simulink model "output_mux_core"  (R2013a)
settings: Solver=ode45  StartTime=0.0  StopTime=10.0  RelTol=1e-3
libraries: xbsIndex_r4 x496, casper_library_misc x1
(part 1 of 2)
settings Model: Creator=jack  LastModifiedBy=jack
settings OptimizationCC: ExpressionDepthLimit=2147483647

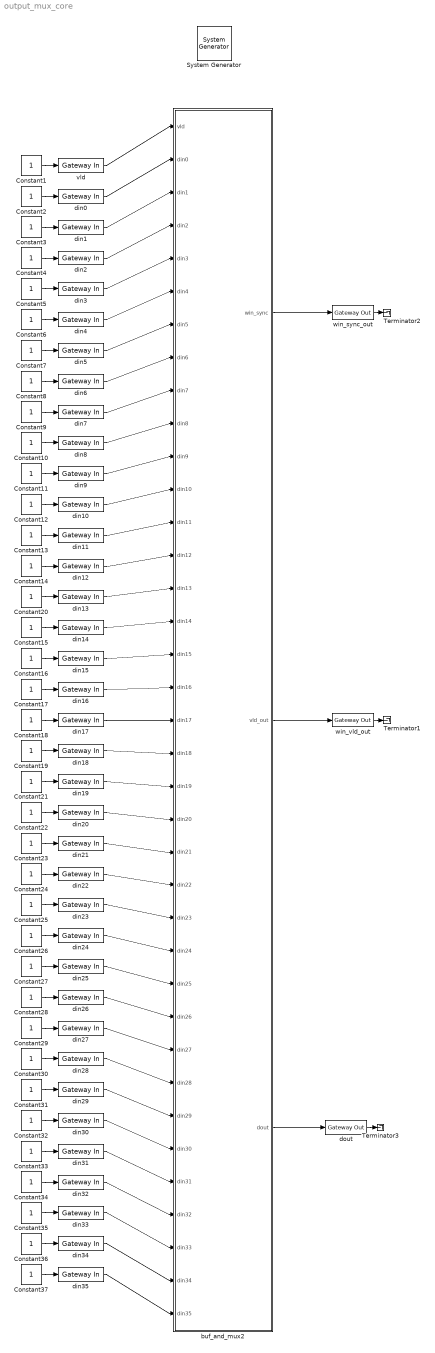
== system output_mux_core ==
  " System Generator" : xbsIndex_r4/ System Generator  Tag=genX  xilinxfamily=virtex6  part=xc6vsx475t  speed=-1  package=ff1759  synthesis_tool=XST  clock_wrapper=Clock Enables  directory=./output_mux_core  proj_type=Project Navigator  Synth_file=XST Defaults  Impl_file=ISE Defaults  testbench=off  simulink_period=1  sysclk_period=3.2  dcm_input_clock_period=10  incr_netlist=off  trim_vbits=Everywhere in SubSystem  dbl_ovrd=According to Block Masks  core_generation=According to Block Masks  run_coregen=off  deprecated_control=off  eval_field=0  block_type=sysgen
  Constant{1..37} (37 alike) : Constant
  Terminator1 : Terminator
  Terminator2 : Terminator
  Terminator3 : Terminator
  buf_and_mux2 : Subsystem  mask{bram_depth=10}
      mask prompts: bram_depth "bram depth (2^?)"
  din{0..35} (36 alike) : xbsIndex_r4/Gateway In  gui_display_data_type=Fixed-point  arith_type=Unsigned  n_bits=64  bin_pt=0  preci_type=Single  exp_width=8  frac_width=24  quantization="Round  (unbiased: +/- Inf)"  overflow=Saturate  period=1  dbl_ovrd=off  timing_constraint=None  locs_specified=off  LOCs={}  UseAsADC=off  ADCChannel='1'  inherit_from_input=off  hdl_port=on  block_type=gatewayin
  dout : xbsIndex_r4/Gateway Out  inherit_from_input=off  hdl_port=on  timing_constraint=None  locs_specified=off  LOCs={}  UseAsDAC=off  DACChannel='1'  block_type=gatewayout
  vld : xbsIndex_r4/Gateway In  gui_display_data_type=Boolean  arith_type=Boolean  n_bits=16  bin_pt=14  preci_type=Single  exp_width=8  frac_width=24  quantization="Round  (unbiased: +/- Inf)"  overflow=Saturate  period=1  dbl_ovrd=off  timing_constraint=None  locs_specified=off  LOCs={}  UseAsADC=off  ADCChannel='1'  inherit_from_input=off  hdl_port=on  block_type=gatewayin
  win_sync_out : xbsIndex_r4/Gateway Out  inherit_from_input=off  hdl_port=on  timing_constraint=None  locs_specified=off  LOCs={}  UseAsDAC=off  DACChannel='1'  block_type=gatewayout
  win_vld_out : xbsIndex_r4/Gateway Out  inherit_from_input=off  hdl_port=on  timing_constraint=None  locs_specified=off  LOCs={}  UseAsDAC=off  DACChannel='1'  block_type=gatewayout
  wires:
  Constant1/1 -> vld/1
  Constant2/1 -> din0/1
  win_sync_out/1 -> Terminator2/1
  vld/1 -> buf_and_mux2/1(vld)
  din0/1 -> buf_and_mux2/2(din0)
  dout/1 -> Terminator3/1
  Constant3/1 -> din1/1
  Constant4/1 -> din2/1
  Constant5/1 -> din3/1
  Constant6/1 -> din4/1
  Constant7/1 -> din5/1
  Constant8/1 -> din6/1
  Constant9/1 -> din7/1
  Constant10/1 -> din8/1
  Constant11/1 -> din9/1
  Constant12/1 -> din10/1
  Constant13/1 -> din11/1
  Constant14/1 -> din12/1
  Constant20/1 -> din13/1
  din5/1 -> buf_and_mux2/7(din5)
  din13/1 -> buf_and_mux2/15(din13)
  din7/1 -> buf_and_mux2/9(din7)
  din3/1 -> buf_and_mux2/5(din3)
  din12/1 -> buf_and_mux2/14(din12)
  din11/1 -> buf_and_mux2/13(din11)
  din4/1 -> buf_and_mux2/6(din4)
  din1/1 -> buf_and_mux2/3(din1)
  din8/1 -> buf_and_mux2/10(din8)
  din10/1 -> buf_and_mux2/12(din10)
  din9/1 -> buf_and_mux2/11(din9)
  din2/1 -> buf_and_mux2/4(din2)
  din6/1 -> buf_and_mux2/8(din6)
  Constant15/1 -> din14/1
  Constant16/1 -> din15/1
  Constant17/1 -> din16/1
  Constant18/1 -> din17/1
  Constant19/1 -> din18/1
  Constant21/1 -> din19/1
  Constant22/1 -> din20/1
  Constant23/1 -> din21/1
  Constant24/1 -> din22/1
  Constant25/1 -> din23/1
  Constant26/1 -> din24/1
  Constant27/1 -> din25/1
  Constant28/1 -> din26/1
  Constant29/1 -> din27/1
  Constant30/1 -> din28/1
  Constant31/1 -> din29/1
  Constant32/1 -> din30/1
  Constant33/1 -> din31/1
  Constant34/1 -> din32/1
  Constant35/1 -> din33/1
  Constant36/1 -> din34/1
  Constant37/1 -> din35/1
  din21/1 -> buf_and_mux2/23(din21)
  din27/1 -> buf_and_mux2/29(din27)
  din31/1 -> buf_and_mux2/33(din31)
  din33/1 -> buf_and_mux2/35(din33)
  din25/1 -> buf_and_mux2/27(din25)
  din34/1 -> buf_and_mux2/36(din34)
  din20/1 -> buf_and_mux2/22(din20)
  din35/1 -> buf_and_mux2/37(din35)
  din24/1 -> buf_and_mux2/26(din24)
  din16/1 -> buf_and_mux2/18(din16)
  din18/1 -> buf_and_mux2/20(din18)
  din23/1 -> buf_and_mux2/25(din23)
  din29/1 -> buf_and_mux2/31(din29)
  din30/1 -> buf_and_mux2/32(din30)
  din19/1 -> buf_and_mux2/21(din19)
  din14/1 -> buf_and_mux2/16(din14)
  din28/1 -> buf_and_mux2/30(din28)
  din17/1 -> buf_and_mux2/19(din17)
  din22/1 -> buf_and_mux2/24(din22)
  din26/1 -> buf_and_mux2/28(din26)
  din15/1 -> buf_and_mux2/17(din15)
  din32/1 -> buf_and_mux2/34(din32)
  buf_and_mux2/1(win_sync) -> win_sync_out/1
  buf_and_mux2/3(dout) -> dout/1
  win_vld_out/1 -> Terminator1/1
  buf_and_mux2/2(vld_out) -> win_vld_out/1

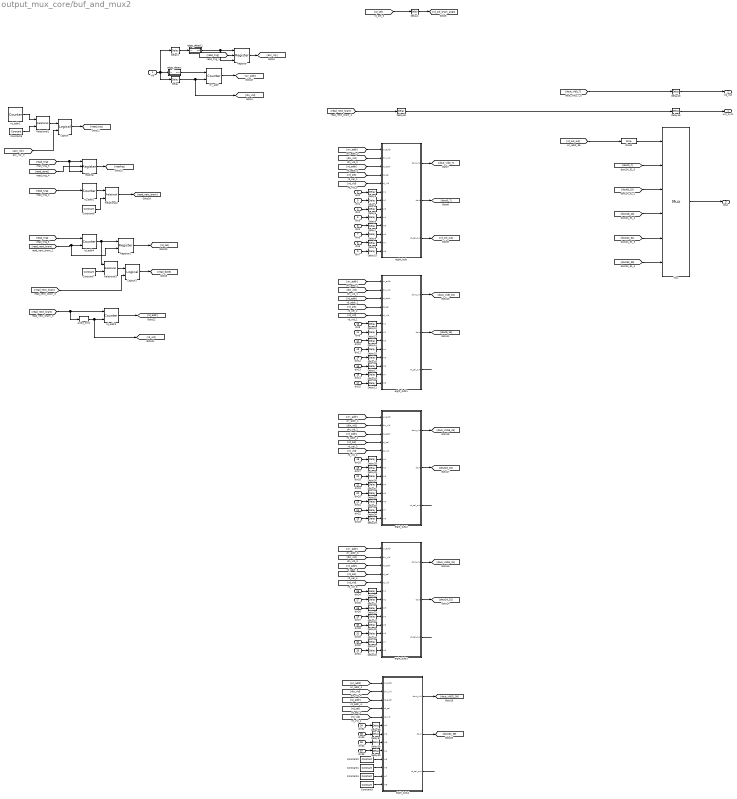
== system output_mux_core/buf_and_mux2 ==
  vld : Inport
  din0 : Inport  Port=2
  din1 : Inport  Port=3
  din2 : Inport  Port=4
  din3 : Inport  Port=5
  din4 : Inport  Port=6
  din5 : Inport  Port=7
  din6 : Inport  Port=8
  din7 : Inport  Port=9
  din8 : Inport  Port=10
  din9 : Inport  Port=11
  din10 : Inport  Port=12
  din11 : Inport  Port=13
  din12 : Inport  Port=14
  din13 : Inport  Port=15
  din14 : Inport  Port=16
  din15 : Inport  Port=17
  din16 : Inport  Port=18
  din17 : Inport  Port=19
  din18 : Inport  Port=20
  din19 : Inport  Port=21
  din20 : Inport  Port=22
  din21 : Inport  Port=23
  din22 : Inport  Port=24
  din23 : Inport  Port=25
  din24 : Inport  Port=26
  din25 : Inport  Port=27
  din26 : Inport  Port=28
  din27 : Inport  Port=29
  din28 : Inport  Port=30
  din29 : Inport  Port=31
  din30 : Inport  Port=32
  din31 : Inport  Port=33
  din32 : Inport  Port=34
  din33 : Inport  Port=35
  din34 : Inport  Port=36
  din35 : Inport  Port=37
  Constant{1..4} (4 alike) : xbsIndex_r4/Constant  const=0  gui_display_data_type=Fixed-point  arith_type=Unsigned  n_bits=64  bin_pt=0  preci_type=Single  exp_width=8  frac_width=24  explicit_period=on  period=1  equ=P=C  opselect=C  inp2=PCIN>>17  opr=+  inp1=P  carry=CIN  dbl_ovrd=off  block_type=constant
  Constant5 : xbsIndex_r4/Constant  const=0  gui_display_data_type=Fixed-point  arith_type=Unsigned  n_bits=bram_depth + 6 + 2  bin_pt=0  preci_type=Single  exp_width=8  frac_width=24  explicit_period=on  period=1  equ=P=C  opselect=C  inp2=PCIN>>17  opr=+  inp1=P  carry=CIN  dbl_ovrd=off  block_type=constant
  Constant6 : xbsIndex_r4/Constant  const=0  gui_display_data_type=Fixed-point  arith_type=Unsigned  n_bits=bram_depth +1  bin_pt=0  preci_type=Single  exp_width=8  frac_width=24  explicit_period=on  period=1  equ=P=C  opselect=C  inp2=PCIN>>17  opr=+  inp1=P  carry=CIN  dbl_ovrd=off  block_type=constant
  Constant7 : xbsIndex_r4/Constant  const=35  gui_display_data_type=Fixed-point  arith_type=Unsigned  n_bits=6  bin_pt=0  preci_type=Single  exp_width=8  frac_width=24  explicit_period=on  period=1  equ=P=C  opselect=C  inp2=PCIN>>17  opr=+  inp1=P  carry=CIN  dbl_ovrd=off  block_type=constant
  Delay{,1,3..34,36..39} (38 alike) : xbsIndex_r4/Delay  rst=off  infoeditControl=Selection of Reset will increase slice count due to use of real FFs and instead of SRLs  en=off  latency=1  dbl_ovrd=off  reg_retiming=off  block_type=delay
  Delay2 : xbsIndex_r4/Delay  rst=off  infoeditControl=Selection of Reset will increase slice count due to use of real FFs and instead of SRLs  en=off  latency=3  dbl_ovrd=off  reg_retiming=off  block_type=delay
  Delay43 : xbsIndex_r4/Delay  rst=off  infoeditControl=Selection of Reset will increase slice count due to use of real FFs and instead of SRLs  en=off  latency=2  dbl_ovrd=off  reg_retiming=off  block_type=delay
  Delay45 : xbsIndex_r4/Delay  rst=off  infoeditControl=Selection of Reset will increase slice count due to use of real FFs and instead of SRLs  en=off  latency=7  dbl_ovrd=off  reg_retiming=on  block_type=delay
  Delay46 : xbsIndex_r4/Delay  rst=off  infoeditControl=Selection of Reset will increase slice count due to use of real FFs and instead of SRLs  en=off  latency=2  dbl_ovrd=off  reg_retiming=off  block_type=delay
  Logical : xbsIndex_r4/Logical  logical_function=AND  inputs=2  en=off  latency=0  precision=Full  arith_type=Unsigned  n_bits=16  bin_pt=0  align_bp=on  dbl_ovrd=off  block_type=logical
  Logical1 : xbsIndex_r4/Logical  logical_function=AND  inputs=2  en=off  latency=0  precision=Full  arith_type=Unsigned  n_bits=16  bin_pt=0  align_bp=on  dbl_ovrd=off  block_type=logical
  Mux : xbsIndex_r4/Mux  inputs=5  en=off  latency=2  precision=Full  arith_type=Unsigned  n_bits=16  bin_pt=14  quantization=Truncate  overflow=Wrap  dbl_ovrd=off  block_type=mux
  Register : xbsIndex_r4/Register  init=0  rst=on  en=on  dbl_ovrd=off  block_type=register
  Register1 : xbsIndex_r4/Register  init=0  rst=off  en=on  dbl_ovrd=off  block_type=register
  Relational1 : xbsIndex_r4/Relational  mode=a=b  en=off  latency=1  dbl_ovrd=off  block_type=relational
  Relational2 : xbsIndex_r4/Relational  mode=a=b  en=off  latency=0  dbl_ovrd=off  block_type=relational
  Relational3 : xbsIndex_r4/Relational  mode=a=b  en=off  latency=0  dbl_ovrd=off  block_type=relational
  Slice2 : xbsIndex_r4/Slice  nbits=3  boolean_output=off  mode=Lower Bit Location + Width  bit1=0  base1=MSB of Input  bit0=3  base0=LSB of Input  dbl_ovrd=off  block_type=slice
  edge_detect : Subsystem  AncestorBlock=casper_library_misc/edge_detect  mask(edge_detect){edge=Rising, polarity=Active High, x_in=[0 0.08 0.08 0.16 0.16 0.24 0.24 0.32 0.32 0.4], y_in=[-1 -1  1  1  1  1  1  1  1  1], x_out=[0.6 0.68 0.68 0.76 0.76 0.84 0.84 0.92 0.92 1], y_out=[-1 -1  1  1 -1 -1 -1 -1 -1 -1]}
      mask prompts: edge "Edge Type"; polarity "Output Polarity"; x_in "Input X Positions"; y_in "Input Y Positions"; x_out "Output X Positions"; y_out "Output Y Positions"
      mask help: Output is active for one-cycle after each edge of the specified type (i.e. rising, falling or both).
      mask init:
      | edge_detect_init(gcb,...
      |     'edge',edge,...
      |     'polarity',polarity,...
      |     'x_in',x_in,...
      |     'x_out',x_out,...
      |     'y_in',y_in,...
      |     'y_out',y_out);
      | 
      | x_in_num=str2num(getfield(getfield(get_param(gcb,'UserData'),'parameters'),'x_in'));
      | x_out_num=str2num(getfield(getfield(get_param(gcb,'UserData'),'parameters'),'x_out'));
      | y_in_num=str2num(getfield(getfield(get_param(gcb,'UserData'),'parameters'),'y_in'));
      | y_out_num=str2num(getfield(getfield(get_param(gcb,'UserData'),'parameters'),'y_out'));
      settings: AttributesFormatString=|
      | rising edges
      | active high
      mask Help: Output is active for one-cycle after each edge of the specified type (i.e. rising, falling, or both).  Latency is zero.
      mask TypeOptions edge: Rising | Falling | Both
      mask TypeOptions polarity: Active High | Active Low
      mask Display:
      | plot(x_in_num,0.5+y_in_num*0.2);
      | plot(x_out_num,0.5+y_out_num*0.2);
  edge_detect1 : Subsystem  AncestorBlock=casper_library_misc/edge_detect  mask(edge_detect){edge=Falling, polarity=Active High, x_in=[0 0.08 0.08 0.16 0.16 0.24 0.24 0.32 0.32 0.4], y_in=[-1 -1  1  1  1  1  1  1  1  1], x_out=[0.6 0.68 0.68 0.76 0.76 0.84 0.84 0.92 0.92 1], y_out=[-1 -1  1  1 -1 -1 -1 -1 -1 -1]}
      mask prompts: edge "Edge Type"; polarity "Output Polarity"; x_in "Input X Positions"; y_in "Input Y Positions"; x_out "Output X Positions"; y_out "Output Y Positions"
      mask help: Output is active for one-cycle after each edge of the specified type (i.e. rising, falling or both).
      mask init: same as output_mux_core/buf_and_mux2/edge_detect
      settings: AttributesFormatString=|
      | falling edges
      | active high
      mask Help: Output is active for one-cycle after each edge of the specified type (i.e. rising, falling, or both).  Latency is zero.
      mask TypeOptions edge: Rising | Falling | Both
      mask TypeOptions polarity: Active High | Active Low
      mask Display:
      | plot(x_in_num,0.5+y_in_num*0.2);
      | plot(x_out_num,0.5+y_out_num*0.2);
  eight_bufs : Subsystem
  eight_bufs1 : Subsystem
  eight_bufs2 : Subsystem
  eight_bufs3 : Subsystem
  eight_bufs4 : Subsystem
  pulse_ext1 : casper_library_misc/pulse_ext  pulse_len=2^bram_depth
  rd_addr1 : xbsIndex_r4/Counter  cnt_type=Free Running  cnt_to=Inf  operation=Up  start_count=0  cnt_by_val=1  arith_type=Unsigned  n_bits=bram_depth + 6 + 2  bin_pt=0  load_pin=off  rst=off  en=off  explicit_period=on  period=1  dbl_ovrd=off  use_behavioral_HDL=off  implementation=Fabric  block_type=counter
  rd_addr2 : xbsIndex_r4/Counter  cnt_type=Count Limited  cnt_to=2^bram_depth  operation=Up  start_count=0  cnt_by_val=1  arith_type=Unsigned  n_bits=bram_depth + 1  bin_pt=0  load_pin=off  rst=on  en=off  explicit_period=on  period=1  dbl_ovrd=off  use_behavioral_HDL=off  implementation=DSP48  block_type=counter
  rd_addr3 : xbsIndex_r4/Counter  cnt_type=Free Running  cnt_to=Inf  operation=Up  start_count=0  cnt_by_val=1  arith_type=Unsigned  n_bits=bram_depth  bin_pt=0  load_pin=off  rst=on  en=on  explicit_period=on  period=1  dbl_ovrd=off  use_behavioral_HDL=off  implementation=Fabric  block_type=counter
  rd_addr4 : xbsIndex_r4/Counter  cnt_type=Free Running  cnt_to=Inf  operation=Up  start_count=0  cnt_by_val=1  arith_type=Unsigned  n_bits=6  bin_pt=0  load_pin=off  rst=on  en=on  explicit_period=on  period=1  dbl_ovrd=off  use_behavioral_HDL=off  implementation=Fabric  block_type=counter
  reading : xbsIndex_r4/Register  init=0  rst=on  en=on  dbl_ovrd=off  block_type=register
  wr_addr : xbsIndex_r4/Counter  cnt_type=Free Running  cnt_to=Inf  operation=Up  start_count=0  cnt_by_val=1  arith_type=Unsigned  n_bits=bram_depth  bin_pt=0  load_pin=off  rst=on  en=on  explicit_period=on  period=1  dbl_ovrd=off  use_behavioral_HDL=off  implementation=DSP48  block_type=counter
  win_sync : Outport
  vld_out : Outport  Port=2
  dout : Outport  Port=3
  wires:
  Register1/1 -> [rd_sel]
  rd_addr4/1 -> Relational3/1, Register1/1
  [read_next_bram] -> rd_addr4/2, Register1/2
  [read_trig] -> rd_addr4/1
  rd_addr3/1 -> [rd_addr]
  pulse_ext1/1 -> rd_addr3/2, [rd_vld]
  [read_next_bram] -> rd_addr3/1, pulse_ext1/1
  [read_done] -> reading/2
  reading/1 -> [reading]
  [read_trig] -> reading/1, reading/3
  Relational2/1 -> [read_next_bram]
  Constant6/1 -> Relational2/2
  rd_addr2/1 -> Relational2/1
  [read_trig] -> rd_addr2/1
  Logical/1 -> [read_trig]
  [acc_rdy] -> Logical/2
  Relational1/1 -> Logical/1
  Constant5/1 -> Relational1/2
  rd_addr1/1 -> Relational1/1
  [read_trig] -> Register/2
  Register/1 -> [acc_rdy]
  Constant4/1 -> eight_bufs4/12(In7)
  Constant3/1 -> eight_bufs4/13(In8)
  Constant1/1 -> eight_bufs4/11(In6)
  Constant2/1 -> eight_bufs4/10(In5)
  Mux/1 -> dout/1
  Delay46/1 -> win_sync/1
  Delay45/1 -> Delay46/1
  [read_next_bram] -> Delay45/1
  Delay43/1 -> vld_out/1
  [dout_vld0_7] -> Delay43/1
  [dout32_39] -> Mux/6
  [dout24_31] -> Mux/5
  [dout8_15] -> Mux/3
  [dout16_23] -> Mux/4
  [dout0_7] -> Mux/2
  eight_bufs4/3(rd_sel_out) -> ?
  eight_bufs4/2(dout) -> [dout32_39]
  eight_bufs4/1(dout_vld) -> [dout_vld32_39]
  Delay39/1 -> eight_bufs4/9(In4)
  Delay38/1 -> eight_bufs4/8(In3)
  Delay37/1 -> eight_bufs4/7(In2)
  Delay36/1 -> eight_bufs4/6(In1)
  [wr_addr] -> eight_bufs4/1(wr_addr)
  [rd_vld] -> eight_bufs4/5(rd_vld)
  [rd_sel] -> eight_bufs4/4(rd_sel)
  [rd_addr] -> eight_bufs4/3(rd_addr)
  [din_vld] -> eight_bufs4/2(din_vld)
  din35/1 -> Delay39/1
  din34/1 -> Delay38/1
  din33/1 -> Delay37/1
  din32/1 -> Delay36/1
  eight_bufs3/3(rd_sel_out) -> ?
  eight_bufs3/2(dout) -> [dout24_31]
  eight_bufs3/1(dout_vld) -> [dout_vld24_31]
  Delay20/1 -> eight_bufs3/13(In8)
  Delay27/1 -> eight_bufs3/12(In7)
  Delay26/1 -> eight_bufs3/11(In6)
  Delay25/1 -> eight_bufs3/10(In5)
  Delay24/1 -> eight_bufs3/9(In4)
  Delay23/1 -> eight_bufs3/8(In3)
  Delay22/1 -> eight_bufs3/7(In2)
  Delay21/1 -> eight_bufs3/6(In1)
  [wr_addr] -> eight_bufs3/1(wr_addr)
  [rd_vld] -> eight_bufs3/5(rd_vld)
  [rd_sel] -> eight_bufs3/4(rd_sel)
  [rd_addr] -> eight_bufs3/3(rd_addr)
  [din_vld] -> eight_bufs3/2(din_vld)
  din31/1 -> Delay20/1
  din30/1 -> Delay27/1
  din29/1 -> Delay26/1
  din28/1 -> Delay25/1
  din27/1 -> Delay24/1
  din26/1 -> Delay23/1
  din25/1 -> Delay22/1
  din24/1 -> Delay21/1
  eight_bufs2/3(rd_sel_out) -> ?
  eight_bufs2/2(dout) -> [dout16_23]
  eight_bufs2/1(dout_vld) -> [dout_vld16_23]
  Delay19/1 -> eight_bufs2/13(In8)
  Delay34/1 -> eight_bufs2/12(In7)
  Delay33/1 -> eight_bufs2/11(In6)
  Delay32/1 -> eight_bufs2/10(In5)
  Delay31/1 -> eight_bufs2/9(In4)
  Delay30/1 -> eight_bufs2/8(In3)
  Delay29/1 -> eight_bufs2/7(In2)
  Delay28/1 -> eight_bufs2/6(In1)
  [wr_addr] -> eight_bufs2/1(wr_addr)
  [rd_vld] -> eight_bufs2/5(rd_vld)
  [rd_sel] -> eight_bufs2/4(rd_sel)
  [rd_addr] -> eight_bufs2/3(rd_addr)
  [din_vld] -> eight_bufs2/2(din_vld)
  din23/1 -> Delay19/1
  din22/1 -> Delay34/1
  din21/1 -> Delay33/1
  din20/1 -> Delay32/1
  din19/1 -> Delay31/1
  din18/1 -> Delay30/1
  din17/1 -> Delay29/1
  din16/1 -> Delay28/1
  eight_bufs1/3(rd_sel_out) -> ?
  eight_bufs1/2(dout) -> [dout8_15]
  eight_bufs1/1(dout_vld) -> [dout_vld8_15]
  Delay11/1 -> eight_bufs1/13(In8)
  Delay18/1 -> eight_bufs1/12(In7)
  Delay17/1 -> eight_bufs1/11(In6)
  Delay16/1 -> eight_bufs1/10(In5)
  Delay15/1 -> eight_bufs1/9(In4)
  Delay14/1 -> eight_bufs1/8(In3)
  Delay13/1 -> eight_bufs1/7(In2)
  Delay12/1 -> eight_bufs1/6(In1)
  [wr_addr] -> eight_bufs1/1(wr_addr)
  [rd_vld] -> eight_bufs1/5(rd_vld)
  [rd_sel] -> eight_bufs1/4(rd_sel)
  [rd_addr] -> eight_bufs1/3(rd_addr)
  [din_vld] -> eight_bufs1/2(din_vld)
  din15/1 -> Delay11/1
  din14/1 -> Delay18/1
  din13/1 -> Delay17/1
  din12/1 -> Delay16/1
  din11/1 -> Delay15/1
  din10/1 -> Delay14/1
  din9/1 -> Delay13/1
  din8/1 -> Delay12/1
  Slice2/1 -> Mux/1
  [rd_sel_out] -> Slice2/1
  eight_bufs/3(rd_sel_out) -> [rd_sel_out]
  eight_bufs/2(dout) -> [dout0_7]
  eight_bufs/1(dout_vld) -> [dout_vld0_7]
  Delay10/1 -> eight_bufs/13(In8)
  Delay9/1 -> eight_bufs/12(In7)
  Delay8/1 -> eight_bufs/11(In6)
  Delay7/1 -> eight_bufs/10(In5)
  Delay6/1 -> eight_bufs/9(In4)
  Delay5/1 -> eight_bufs/8(In3)
  Delay4/1 -> eight_bufs/7(In2)
  Delay3/1 -> eight_bufs/6(In1)
  [wr_addr] -> eight_bufs/1(wr_addr)
  [rd_vld] -> eight_bufs/5(rd_vld)
  [rd_sel] -> eight_bufs/4(rd_sel)
  [rd_addr] -> eight_bufs/3(rd_addr)
  [din_vld] -> eight_bufs/2(din_vld)
  din7/1 -> Delay10/1
  din6/1 -> Delay9/1
  din5/1 -> Delay8/1
  din4/1 -> Delay7/1
  din3/1 -> Delay6/1
  din2/1 -> Delay5/1
  din1/1 -> Delay4/1
  din0/1 -> Delay3/1
  Delay2/1 -> [rd_sel_bram_align]
  [rd_sel] -> Delay2/1
  Delay1/1 -> edge_detect1/1(in)
  edge_detect1/1(out) -> Register/1, Register/3
  wr_addr/1 -> [wr_addr]
  Delay/1 -> wr_addr/2, [din_vld]
  edge_detect/1(out) -> wr_addr/1
  vld/1 -> edge_detect/1(in), Delay/1, Delay1/1
  Constant7/1 -> Relational3/2
  Relational3/1 -> Logical1/1
  [read_next_bram] -> Logical1/2
  Logical1/1 -> [read_done]

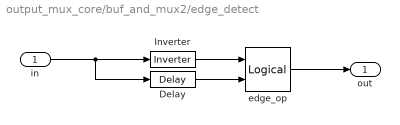
== system output_mux_core/buf_and_mux2/edge_detect ==
  in : Inport
  Delay : xbsIndex_r4/Delay  rst=off  infoeditControl=Selection of Reset will increase slice count due to use of real FFs and instead of SRLs  en=off  latency=1  dbl_ovrd=off  reg_retiming=off  block_type=delay
      settings: xl_area=[0, 0, 0, 0, 0, 0, 0]
  Inverter : xbsIndex_r4/Inverter  en=off  latency=0  dbl_ovrd=off  block_type=inv
      settings: xl_area=[0, 0, 0, 0, 0, 0, 0]
  edge_op : xbsIndex_r4/Logical  logical_function=NOR  inputs=2  en=off  latency=0  precision=Full  arith_type=Unsigned  n_bits=8  bin_pt=2  align_bp=on  dbl_ovrd=off  block_type=logical
      settings: xl_area=[0, 0, 0, 0, 0, 0, 0]
  out : Outport
  wires:
  Delay/1 -> edge_op/2
  in/1 -> Delay/1, Inverter/1
  edge_op/1 -> out/1
  Inverter/1 -> edge_op/1

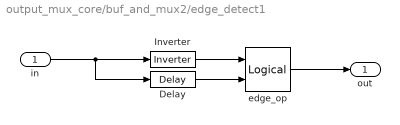
== system output_mux_core/buf_and_mux2/edge_detect1 ==
  in : Inport
  Delay : xbsIndex_r4/Delay  rst=off  infoeditControl=Selection of Reset will increase slice count due to use of real FFs and instead of SRLs  en=off  latency=1  dbl_ovrd=off  reg_retiming=off  block_type=delay
      settings: xl_area=[0, 0, 0, 0, 0, 0, 0]
  Inverter : xbsIndex_r4/Inverter  en=off  latency=0  dbl_ovrd=off  block_type=inv
      settings: xl_area=[0, 0, 0, 0, 0, 0, 0]
  edge_op : xbsIndex_r4/Logical  logical_function=AND  inputs=2  en=off  latency=0  precision=Full  arith_type=Unsigned  n_bits=8  bin_pt=2  align_bp=on  dbl_ovrd=off  block_type=logical
      settings: xl_area=[0, 0, 0, 0, 0, 0, 0]
  out : Outport
  wires:
  Inverter/1 -> edge_op/1
  edge_op/1 -> out/1
  in/1 -> Inverter/1, Delay/1
  Delay/1 -> edge_op/2

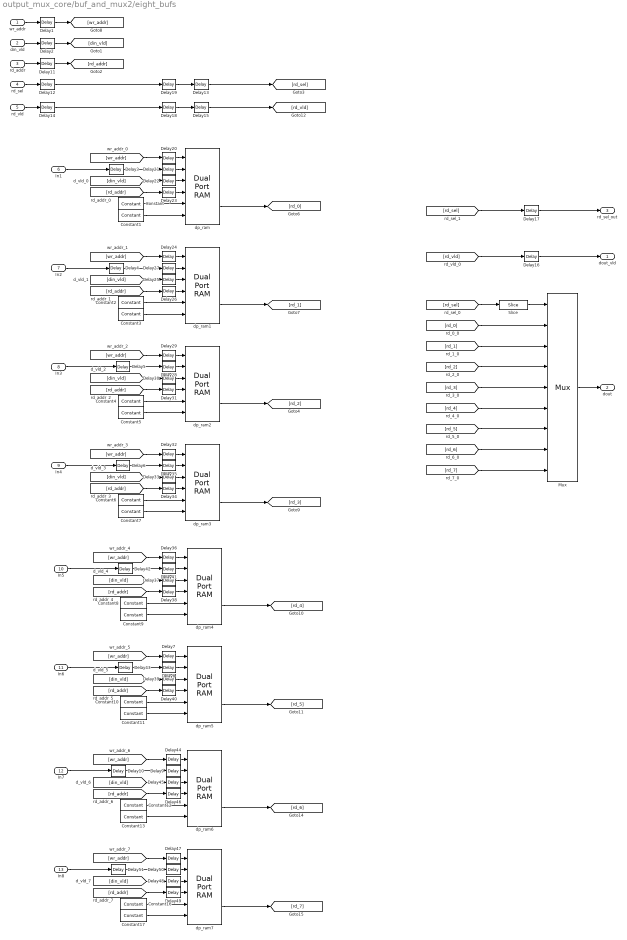
== system output_mux_core/buf_and_mux2/eight_bufs ==
  wr_addr : Inport
  din_vld : Inport  Port=2
  rd_addr : Inport  Port=3
  rd_sel : Inport  Port=4
  rd_vld : Inport  Port=5
  In1 : Inport  Port=6
  In2 : Inport  Port=7
  In3 : Inport  Port=8
  In4 : Inport  Port=9
  In5 : Inport  Port=10
  In6 : Inport  Port=11
  In7 : Inport  Port=12
  In8 : Inport  Port=13
  Constant{,2,4,6,8,10,12,16} (8 alike) : xbsIndex_r4/Constant  const=0  gui_display_data_type=Fixed-point  arith_type=Unsigned  n_bits=64  bin_pt=0  preci_type=Single  exp_width=8  frac_width=24  explicit_period=on  period=1  equ=P=C  opselect=C  inp2=PCIN>>17  opr=+  inp1=P  carry=CIN  dbl_ovrd=off  block_type=constant
  Constant{1,3,5,7,9,11,13,17} (8 alike) : xbsIndex_r4/Constant  const=0  gui_display_data_type=Boolean  arith_type=Boolean  n_bits=64  bin_pt=0  preci_type=Single  exp_width=8  frac_width=24  explicit_period=on  period=1  equ=P=C  opselect=C  inp2=PCIN>>17  opr=+  inp1=P  carry=CIN  dbl_ovrd=off  block_type=constant
  Delay{1..2,7,11..12,14,20,22..26,29..34,36..40,44..49} (29 alike) : xbsIndex_r4/Delay  rst=off  infoeditControl=Selection of Reset will increase slice count due to use of real FFs and instead of SRLs  en=off  latency=1  dbl_ovrd=off  reg_retiming=off  block_type=delay
  Delay{3..6,8..10,18..19,21,27..28,35,41..43,50..51} (18 alike) : xbsIndex_r4/Delay  rst=off  infoeditControl=Selection of Reset will increase slice count due to use of real FFs and instead of SRLs  en=off  latency=1  dbl_ovrd=off  reg_retiming=on  block_type=delay
  Delay13 : xbsIndex_r4/Delay  rst=off  infoeditControl=Selection of Reset will increase slice count due to use of real FFs and instead of SRLs  en=off  latency=3  dbl_ovrd=off  reg_retiming=on  block_type=delay
  Delay15 : xbsIndex_r4/Delay  rst=off  infoeditControl=Selection of Reset will increase slice count due to use of real FFs and instead of SRLs  en=off  latency=3  dbl_ovrd=off  reg_retiming=on  block_type=delay
  Delay16 : xbsIndex_r4/Delay  rst=off  infoeditControl=Selection of Reset will increase slice count due to use of real FFs and instead of SRLs  en=off  latency=2  dbl_ovrd=off  reg_retiming=off  block_type=delay
  Delay17 : xbsIndex_r4/Delay  rst=off  infoeditControl=Selection of Reset will increase slice count due to use of real FFs and instead of SRLs  en=off  latency=2  dbl_ovrd=off  reg_retiming=off  block_type=delay
  Mux : xbsIndex_r4/Mux  inputs=8  en=off  latency=2  precision=Full  arith_type=Unsigned  n_bits=16  bin_pt=14  quantization=Truncate  overflow=Wrap  dbl_ovrd=off  block_type=mux
  Slice : xbsIndex_r4/Slice  nbits=3  boolean_output=off  mode=Lower Bit Location + Width  bit1=0  base1=MSB of Input  bit0=0  base0=LSB of Input  dbl_ovrd=off  block_type=slice
  dp_ram{,1..7} (8 alike) : xbsIndex_r4/Dual Port RAM  depth=2^bram_depth  initVector=sin(pi*(0:15)/16)  distributed_mem=Block RAM  init_a=0  init_b=0  rst_a=off  rst_b=off  en_a=off  en_b=off  latency=3  write_mode_A=Read After Write  write_mode_B=Read After Write  dbl_ovrd=off  optimize=Speed  block_type=dpram
  dout_vld : Outport
  dout : Outport  Port=2
  rd_sel_out : Outport  Port=3
  wires:
  Slice/1 -> Mux/1
  Delay17/1 -> rd_sel_out/1
  [rd_sel] -> Delay17/1
  Delay16/1 -> dout_vld/1
  [rd_vld] -> Delay16/1
  Delay14/1 -> Delay18/1
  Delay15/1 -> [rd_vld]
  rd_vld/1 -> Delay14/1
  Mux/1 -> dout/1
  [rd_1] -> Mux/3
  [rd_2] -> Mux/4
  [rd_0] -> Mux/2
  [rd_5] -> Mux/7
  [rd_4] -> Mux/6
  [rd_sel] -> Slice/1
  [rd_7] -> Mux/9
  [rd_6] -> Mux/8
  [rd_3] -> Mux/5
  dp_ram7/2 -> [rd_7]
  dp_ram6/2 -> [rd_6]
  dp_ram5/2 -> [rd_5]
  dp_ram4/2 -> [rd_4]
  dp_ram3/2 -> [rd_3]
  dp_ram2/2 -> [rd_2]
  dp_ram1/2 -> [rd_1]
  dp_ram/2 -> [rd_0]
  Delay13/1 -> [rd_sel]
  Delay12/1 -> Delay19/1
  rd_sel/1 -> Delay12/1
  Delay11/1 -> [rd_addr]
  rd_addr/1 -> Delay11/1
  Delay2/1 -> [din_vld]
  din_vld/1 -> Delay2/1
  Delay1/1 -> [wr_addr]
  wr_addr/1 -> Delay1/1
  Constant1/1 -> dp_ram/6
  [wr_addr] -> Delay44/1
  Constant17/1 -> dp_ram7/6
  [wr_addr] -> Delay7/1
  [din_vld] -> Delay22/1
  [din_vld] -> Delay39/1
  Delay4/1 -> Delay27/1
  Delay51/1 -> Delay50/1
  [rd_addr] -> Delay46/1
  Constant7/1 -> dp_ram3/6
  In4/1 -> Delay6/1
  Constant11/1 -> dp_ram5/6
  Constant13/1 -> dp_ram6/6
  Delay42/1 -> Delay41/1
  [din_vld] -> Delay33/1
  Constant10/1 -> dp_ram5/5
  [rd_addr] -> Delay38/1
  Constant4/1 -> dp_ram2/5
  Constant12/1 -> dp_ram6/5
  Constant8/1 -> dp_ram4/5
  [din_vld] -> Delay30/1
  Delay43/1 -> Delay8/1
  [din_vld] -> Delay48/1
  [din_vld] -> Delay37/1
  [rd_addr] -> Delay40/1
  In1/1 -> Delay3/1
  [rd_addr] -> Delay34/1
  Delay10/1 -> Delay9/1
  [rd_addr] -> Delay31/1
  Delay5/1 -> Delay28/1
  [wr_addr] -> Delay47/1
  Constant16/1 -> dp_ram7/5
  In6/1 -> Delay43/1
  Constant6/1 -> dp_ram3/5
  Constant9/1 -> dp_ram4/6
  In3/1 -> Delay5/1
  In8/1 -> Delay51/1
  [wr_addr] -> Delay36/1
  [wr_addr] -> Delay29/1
  In7/1 -> Delay10/1
  Constant/1 -> dp_ram/5
  Constant5/1 -> dp_ram2/6
  [rd_addr] -> Delay49/1
  In5/1 -> Delay42/1
  [wr_addr] -> Delay32/1
  [wr_addr] -> Delay20/1
  [wr_addr] -> Delay24/1
  [rd_addr] -> Delay26/1
  In2/1 -> Delay4/1
  Constant2/1 -> dp_ram1/5
  Constant3/1 -> dp_ram1/6
  [din_vld] -> Delay25/1
  [din_vld] -> Delay45/1
  [rd_addr] -> Delay23/1
  Delay3/1 -> Delay21/1
  Delay18/1 -> Delay15/1
  Delay19/1 -> Delay13/1
  Delay20/1 -> dp_ram/1
  Delay21/1 -> dp_ram/2
  Delay22/1 -> dp_ram/3
  Delay23/1 -> dp_ram/4
  Delay24/1 -> dp_ram1/1
  Delay25/1 -> dp_ram1/3
  Delay26/1 -> dp_ram1/4
  Delay27/1 -> dp_ram1/2
  Delay28/1 -> dp_ram2/2
  Delay29/1 -> dp_ram2/1
  Delay30/1 -> dp_ram2/3
  Delay31/1 -> dp_ram2/4
  Delay32/1 -> dp_ram3/1
  Delay33/1 -> dp_ram3/3
  Delay34/1 -> dp_ram3/4
  Delay6/1 -> Delay35/1
  Delay35/1 -> dp_ram3/2
  Delay36/1 -> dp_ram4/1
  Delay37/1 -> dp_ram4/3
  Delay38/1 -> dp_ram4/4
  Delay7/1 -> dp_ram5/1
  Delay39/1 -> dp_ram5/3
  Delay40/1 -> dp_ram5/4
  Delay41/1 -> dp_ram4/2
  Delay8/1 -> dp_ram5/2
  Delay44/1 -> dp_ram6/1
  Delay45/1 -> dp_ram6/3
  Delay46/1 -> dp_ram6/4
  Delay47/1 -> dp_ram7/1
  Delay48/1 -> dp_ram7/3
  Delay49/1 -> dp_ram7/4
  Delay9/1 -> dp_ram6/2
  Delay50/1 -> dp_ram7/2

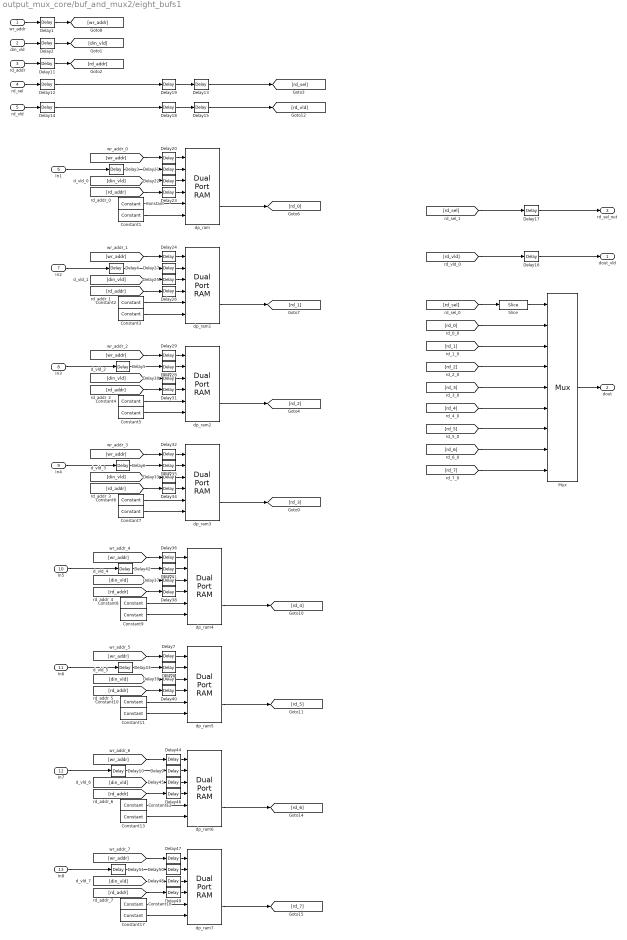
== system output_mux_core/buf_and_mux2/eight_bufs1 ==
  wr_addr : Inport
  din_vld : Inport  Port=2
  rd_addr : Inport  Port=3
  rd_sel : Inport  Port=4
  rd_vld : Inport  Port=5
  In1 : Inport  Port=6
  In2 : Inport  Port=7
  In3 : Inport  Port=8
  In4 : Inport  Port=9
  In5 : Inport  Port=10
  In6 : Inport  Port=11
  In7 : Inport  Port=12
  In8 : Inport  Port=13
  Constant{,2,4,6,8,10,12,16} (8 alike) : xbsIndex_r4/Constant  const=0  gui_display_data_type=Fixed-point  arith_type=Unsigned  n_bits=64  bin_pt=0  preci_type=Single  exp_width=8  frac_width=24  explicit_period=on  period=1  equ=P=C  opselect=C  inp2=PCIN>>17  opr=+  inp1=P  carry=CIN  dbl_ovrd=off  block_type=constant
  Constant{1,3,5,7,9,11,13,17} (8 alike) : xbsIndex_r4/Constant  const=0  gui_display_data_type=Boolean  arith_type=Boolean  n_bits=64  bin_pt=0  preci_type=Single  exp_width=8  frac_width=24  explicit_period=on  period=1  equ=P=C  opselect=C  inp2=PCIN>>17  opr=+  inp1=P  carry=CIN  dbl_ovrd=off  block_type=constant
  Delay{1..2,7,11..12,14,20,22..26,29..34,36..40,44..49} (29 alike) : xbsIndex_r4/Delay  rst=off  infoeditControl=Selection of Reset will increase slice count due to use of real FFs and instead of SRLs  en=off  latency=1  dbl_ovrd=off  reg_retiming=off  block_type=delay
  Delay{3..6,8..10,18..19,21,27..28,35,41..43,50..51} (18 alike) : xbsIndex_r4/Delay  rst=off  infoeditControl=Selection of Reset will increase slice count due to use of real FFs and instead of SRLs  en=off  latency=1  dbl_ovrd=off  reg_retiming=on  block_type=delay
  Delay13 : xbsIndex_r4/Delay  rst=off  infoeditControl=Selection of Reset will increase slice count due to use of real FFs and instead of SRLs  en=off  latency=3  dbl_ovrd=off  reg_retiming=on  block_type=delay
  Delay15 : xbsIndex_r4/Delay  rst=off  infoeditControl=Selection of Reset will increase slice count due to use of real FFs and instead of SRLs  en=off  latency=3  dbl_ovrd=off  reg_retiming=on  block_type=delay
  Delay16 : xbsIndex_r4/Delay  rst=off  infoeditControl=Selection of Reset will increase slice count due to use of real FFs and instead of SRLs  en=off  latency=2  dbl_ovrd=off  reg_retiming=off  block_type=delay
  Delay17 : xbsIndex_r4/Delay  rst=off  infoeditControl=Selection of Reset will increase slice count due to use of real FFs and instead of SRLs  en=off  latency=2  dbl_ovrd=off  reg_retiming=off  block_type=delay
  Mux : xbsIndex_r4/Mux  inputs=8  en=off  latency=2  precision=Full  arith_type=Unsigned  n_bits=16  bin_pt=14  quantization=Truncate  overflow=Wrap  dbl_ovrd=off  block_type=mux
  Slice : xbsIndex_r4/Slice  nbits=3  boolean_output=off  mode=Lower Bit Location + Width  bit1=0  base1=MSB of Input  bit0=0  base0=LSB of Input  dbl_ovrd=off  block_type=slice
  dp_ram{,1..7} (8 alike) : xbsIndex_r4/Dual Port RAM  depth=2^bram_depth  initVector=sin(pi*(0:15)/16)  distributed_mem=Block RAM  init_a=0  init_b=0  rst_a=off  rst_b=off  en_a=off  en_b=off  latency=3  write_mode_A=Read After Write  write_mode_B=Read After Write  dbl_ovrd=off  optimize=Speed  block_type=dpram
  dout_vld : Outport
  dout : Outport  Port=2
  rd_sel_out : Outport  Port=3
  wires:
  Delay50/1 -> dp_ram7/2
  Delay9/1 -> dp_ram6/2
  Delay49/1 -> dp_ram7/4
  Delay48/1 -> dp_ram7/3
  Delay47/1 -> dp_ram7/1
  Delay46/1 -> dp_ram6/4
  Delay45/1 -> dp_ram6/3
  Delay44/1 -> dp_ram6/1
  Delay8/1 -> dp_ram5/2
  Delay41/1 -> dp_ram4/2
  Delay40/1 -> dp_ram5/4
  Delay39/1 -> dp_ram5/3
  Delay7/1 -> dp_ram5/1
  Delay38/1 -> dp_ram4/4
  Delay37/1 -> dp_ram4/3
  Delay36/1 -> dp_ram4/1
  Delay35/1 -> dp_ram3/2
  Delay6/1 -> Delay35/1
  Delay34/1 -> dp_ram3/4
  Delay33/1 -> dp_ram3/3
  Delay32/1 -> dp_ram3/1
  Delay31/1 -> dp_ram2/4
  Delay30/1 -> dp_ram2/3
  Delay29/1 -> dp_ram2/1
  Delay28/1 -> dp_ram2/2
  Delay27/1 -> dp_ram1/2
  Delay26/1 -> dp_ram1/4
  Delay25/1 -> dp_ram1/3
  Delay24/1 -> dp_ram1/1
  Delay23/1 -> dp_ram/4
  Delay22/1 -> dp_ram/3
  Delay21/1 -> dp_ram/2
  Delay20/1 -> dp_ram/1
  Delay19/1 -> Delay13/1
  Delay18/1 -> Delay15/1
  Delay3/1 -> Delay21/1
  [rd_addr] -> Delay23/1
  [din_vld] -> Delay45/1
  [din_vld] -> Delay25/1
  Constant3/1 -> dp_ram1/6
  Constant2/1 -> dp_ram1/5
  In2/1 -> Delay4/1
  [rd_addr] -> Delay26/1
  [wr_addr] -> Delay24/1
  [wr_addr] -> Delay20/1
  [wr_addr] -> Delay32/1
  In5/1 -> Delay42/1
  [rd_addr] -> Delay49/1
  Constant5/1 -> dp_ram2/6
  Constant/1 -> dp_ram/5
  In7/1 -> Delay10/1
  [wr_addr] -> Delay29/1
  [wr_addr] -> Delay36/1
  In8/1 -> Delay51/1
  In3/1 -> Delay5/1
  Constant9/1 -> dp_ram4/6
  Constant6/1 -> dp_ram3/5
  In6/1 -> Delay43/1
  Constant16/1 -> dp_ram7/5
  [wr_addr] -> Delay47/1
  Delay5/1 -> Delay28/1
  [rd_addr] -> Delay31/1
  Delay10/1 -> Delay9/1
  [rd_addr] -> Delay34/1
  In1/1 -> Delay3/1
  [rd_addr] -> Delay40/1
  [din_vld] -> Delay37/1
  [din_vld] -> Delay48/1
  Delay43/1 -> Delay8/1
  [din_vld] -> Delay30/1
  Constant8/1 -> dp_ram4/5
  Constant12/1 -> dp_ram6/5
  Constant4/1 -> dp_ram2/5
  [rd_addr] -> Delay38/1
  Constant10/1 -> dp_ram5/5
  [din_vld] -> Delay33/1
  Delay42/1 -> Delay41/1
  Constant13/1 -> dp_ram6/6
  Constant11/1 -> dp_ram5/6
  In4/1 -> Delay6/1
  Constant7/1 -> dp_ram3/6
  [rd_addr] -> Delay46/1
  Delay51/1 -> Delay50/1
  Delay4/1 -> Delay27/1
  [din_vld] -> Delay39/1
  [din_vld] -> Delay22/1
  [wr_addr] -> Delay7/1
  Constant17/1 -> dp_ram7/6
  [wr_addr] -> Delay44/1
  Constant1/1 -> dp_ram/6
  wr_addr/1 -> Delay1/1
  Delay1/1 -> [wr_addr]
  din_vld/1 -> Delay2/1
  Delay2/1 -> [din_vld]
  rd_addr/1 -> Delay11/1
  Delay11/1 -> [rd_addr]
  rd_sel/1 -> Delay12/1
  Delay12/1 -> Delay19/1
  Delay13/1 -> [rd_sel]
  dp_ram/2 -> [rd_0]
  dp_ram1/2 -> [rd_1]
  dp_ram2/2 -> [rd_2]
  dp_ram3/2 -> [rd_3]
  dp_ram4/2 -> [rd_4]
  dp_ram5/2 -> [rd_5]
  dp_ram6/2 -> [rd_6]
  dp_ram7/2 -> [rd_7]
  [rd_3] -> Mux/5
  [rd_6] -> Mux/8
  [rd_7] -> Mux/9
  [rd_sel] -> Slice/1
  [rd_4] -> Mux/6
  [rd_5] -> Mux/7
  [rd_0] -> Mux/2
  [rd_2] -> Mux/4
  [rd_1] -> Mux/3
  Mux/1 -> dout/1
  rd_vld/1 -> Delay14/1
  Delay15/1 -> [rd_vld]
  Delay14/1 -> Delay18/1
  [rd_vld] -> Delay16/1
  Delay16/1 -> dout_vld/1
  [rd_sel] -> Delay17/1
  Delay17/1 -> rd_sel_out/1
  Slice/1 -> Mux/1

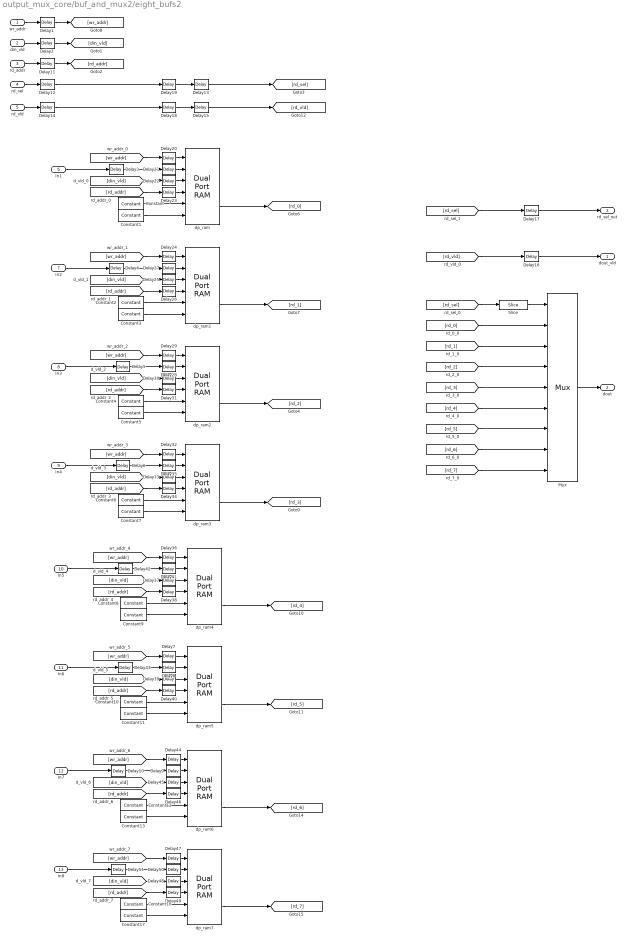
== system output_mux_core/buf_and_mux2/eight_bufs2 ==
  wr_addr : Inport
  din_vld : Inport  Port=2
  rd_addr : Inport  Port=3
  rd_sel : Inport  Port=4
  rd_vld : Inport  Port=5
  In1 : Inport  Port=6
  In2 : Inport  Port=7
  In3 : Inport  Port=8
  In4 : Inport  Port=9
  In5 : Inport  Port=10
  In6 : Inport  Port=11
  In7 : Inport  Port=12
  In8 : Inport  Port=13
  Constant{,2,4,6,8,10,12,16} (8 alike) : xbsIndex_r4/Constant  const=0  gui_display_data_type=Fixed-point  arith_type=Unsigned  n_bits=64  bin_pt=0  preci_type=Single  exp_width=8  frac_width=24  explicit_period=on  period=1  equ=P=C  opselect=C  inp2=PCIN>>17  opr=+  inp1=P  carry=CIN  dbl_ovrd=off  block_type=constant
  Constant{1,3,5,7,9,11,13,17} (8 alike) : xbsIndex_r4/Constant  const=0  gui_display_data_type=Boolean  arith_type=Boolean  n_bits=64  bin_pt=0  preci_type=Single  exp_width=8  frac_width=24  explicit_period=on  period=1  equ=P=C  opselect=C  inp2=PCIN>>17  opr=+  inp1=P  carry=CIN  dbl_ovrd=off  block_type=constant
  Delay{1..2,7,11..12,14,20,22..26,29..34,36..40,44..49} (29 alike) : xbsIndex_r4/Delay  rst=off  infoeditControl=Selection of Reset will increase slice count due to use of real FFs and instead of SRLs  en=off  latency=1  dbl_ovrd=off  reg_retiming=off  block_type=delay
  Delay{3..6,8..10,18..19,21,27..28,35,41..43,50..51} (18 alike) : xbsIndex_r4/Delay  rst=off  infoeditControl=Selection of Reset will increase slice count due to use of real FFs and instead of SRLs  en=off  latency=1  dbl_ovrd=off  reg_retiming=on  block_type=delay
  Delay13 : xbsIndex_r4/Delay  rst=off  infoeditControl=Selection of Reset will increase slice count due to use of real FFs and instead of SRLs  en=off  latency=3  dbl_ovrd=off  reg_retiming=on  block_type=delay
  Delay15 : xbsIndex_r4/Delay  rst=off  infoeditControl=Selection of Reset will increase slice count due to use of real FFs and instead of SRLs  en=off  latency=3  dbl_ovrd=off  reg_retiming=on  block_type=delay
  Delay16 : xbsIndex_r4/Delay  rst=off  infoeditControl=Selection of Reset will increase slice count due to use of real FFs and instead of SRLs  en=off  latency=2  dbl_ovrd=off  reg_retiming=off  block_type=delay
  Delay17 : xbsIndex_r4/Delay  rst=off  infoeditControl=Selection of Reset will increase slice count due to use of real FFs and instead of SRLs  en=off  latency=2  dbl_ovrd=off  reg_retiming=off  block_type=delay
  Mux : xbsIndex_r4/Mux  inputs=8  en=off  latency=2  precision=Full  arith_type=Unsigned  n_bits=16  bin_pt=14  quantization=Truncate  overflow=Wrap  dbl_ovrd=off  block_type=mux
  Slice : xbsIndex_r4/Slice  nbits=3  boolean_output=off  mode=Lower Bit Location + Width  bit1=0  base1=MSB of Input  bit0=0  base0=LSB of Input  dbl_ovrd=off  block_type=slice
  dp_ram{,1..7} (8 alike) : xbsIndex_r4/Dual Port RAM  depth=2^bram_depth  initVector=sin(pi*(0:15)/16)  distributed_mem=Block RAM  init_a=0  init_b=0  rst_a=off  rst_b=off  en_a=off  en_b=off  latency=3  write_mode_A=Read After Write  write_mode_B=Read After Write  dbl_ovrd=off  optimize=Speed  block_type=dpram
  dout_vld : Outport
  dout : Outport  Port=2
  rd_sel_out : Outport  Port=3
  wires:
  Slice/1 -> Mux/1
  Delay17/1 -> rd_sel_out/1
  [rd_sel] -> Delay17/1
  Delay16/1 -> dout_vld/1
  [rd_vld] -> Delay16/1
  Delay14/1 -> Delay18/1
  Delay15/1 -> [rd_vld]
  rd_vld/1 -> Delay14/1
  Mux/1 -> dout/1
  [rd_1] -> Mux/3
  [rd_2] -> Mux/4
  [rd_0] -> Mux/2
  [rd_5] -> Mux/7
  [rd_4] -> Mux/6
  [rd_sel] -> Slice/1
  [rd_7] -> Mux/9
  [rd_6] -> Mux/8
  [rd_3] -> Mux/5
  dp_ram7/2 -> [rd_7]
  dp_ram6/2 -> [rd_6]
  dp_ram5/2 -> [rd_5]
  dp_ram4/2 -> [rd_4]
  dp_ram3/2 -> [rd_3]
  dp_ram2/2 -> [rd_2]
  dp_ram1/2 -> [rd_1]
  dp_ram/2 -> [rd_0]
  Delay13/1 -> [rd_sel]
  Delay12/1 -> Delay19/1
  rd_sel/1 -> Delay12/1
  Delay11/1 -> [rd_addr]
  rd_addr/1 -> Delay11/1
  Delay2/1 -> [din_vld]
  din_vld/1 -> Delay2/1
  Delay1/1 -> [wr_addr]
  wr_addr/1 -> Delay1/1
  Constant1/1 -> dp_ram/6
  [wr_addr] -> Delay44/1
  Constant17/1 -> dp_ram7/6
  [wr_addr] -> Delay7/1
  [din_vld] -> Delay22/1
  [din_vld] -> Delay39/1
  Delay4/1 -> Delay27/1
  Delay51/1 -> Delay50/1
  [rd_addr] -> Delay46/1
  Constant7/1 -> dp_ram3/6
  In4/1 -> Delay6/1
  Constant11/1 -> dp_ram5/6
  Constant13/1 -> dp_ram6/6
  Delay42/1 -> Delay41/1
  [din_vld] -> Delay33/1
  Constant10/1 -> dp_ram5/5
  [rd_addr] -> Delay38/1
  Constant4/1 -> dp_ram2/5
  Constant12/1 -> dp_ram6/5
  Constant8/1 -> dp_ram4/5
  [din_vld] -> Delay30/1
  Delay43/1 -> Delay8/1
  [din_vld] -> Delay48/1
  [din_vld] -> Delay37/1
  [rd_addr] -> Delay40/1
  In1/1 -> Delay3/1
  [rd_addr] -> Delay34/1
  Delay10/1 -> Delay9/1
  [rd_addr] -> Delay31/1
  Delay5/1 -> Delay28/1
  [wr_addr] -> Delay47/1
  Constant16/1 -> dp_ram7/5
  In6/1 -> Delay43/1
  Constant6/1 -> dp_ram3/5
  Constant9/1 -> dp_ram4/6
  In3/1 -> Delay5/1
  In8/1 -> Delay51/1
  [wr_addr] -> Delay36/1
  [wr_addr] -> Delay29/1
  In7/1 -> Delay10/1
  Constant/1 -> dp_ram/5
  Constant5/1 -> dp_ram2/6
  [rd_addr] -> Delay49/1
  In5/1 -> Delay42/1
  [wr_addr] -> Delay32/1
  [wr_addr] -> Delay20/1
  [wr_addr] -> Delay24/1
  [rd_addr] -> Delay26/1
  In2/1 -> Delay4/1
  Constant2/1 -> dp_ram1/5
  Constant3/1 -> dp_ram1/6
  [din_vld] -> Delay25/1
  [din_vld] -> Delay45/1
  [rd_addr] -> Delay23/1
  Delay3/1 -> Delay21/1
  Delay18/1 -> Delay15/1
  Delay19/1 -> Delay13/1
  Delay20/1 -> dp_ram/1
  Delay21/1 -> dp_ram/2
  Delay22/1 -> dp_ram/3
  Delay23/1 -> dp_ram/4
  Delay24/1 -> dp_ram1/1
  Delay25/1 -> dp_ram1/3
  Delay26/1 -> dp_ram1/4
  Delay27/1 -> dp_ram1/2
  Delay28/1 -> dp_ram2/2
  Delay29/1 -> dp_ram2/1
  Delay30/1 -> dp_ram2/3
  Delay31/1 -> dp_ram2/4
  Delay32/1 -> dp_ram3/1
  Delay33/1 -> dp_ram3/3
  Delay34/1 -> dp_ram3/4
  Delay6/1 -> Delay35/1
  Delay35/1 -> dp_ram3/2
  Delay36/1 -> dp_ram4/1
  Delay37/1 -> dp_ram4/3
  Delay38/1 -> dp_ram4/4
  Delay7/1 -> dp_ram5/1
  Delay39/1 -> dp_ram5/3
  Delay40/1 -> dp_ram5/4
  Delay41/1 -> dp_ram4/2
  Delay8/1 -> dp_ram5/2
  Delay44/1 -> dp_ram6/1
  Delay45/1 -> dp_ram6/3
  Delay46/1 -> dp_ram6/4
  Delay47/1 -> dp_ram7/1
  Delay48/1 -> dp_ram7/3
  Delay49/1 -> dp_ram7/4
  Delay9/1 -> dp_ram6/2
  Delay50/1 -> dp_ram7/2

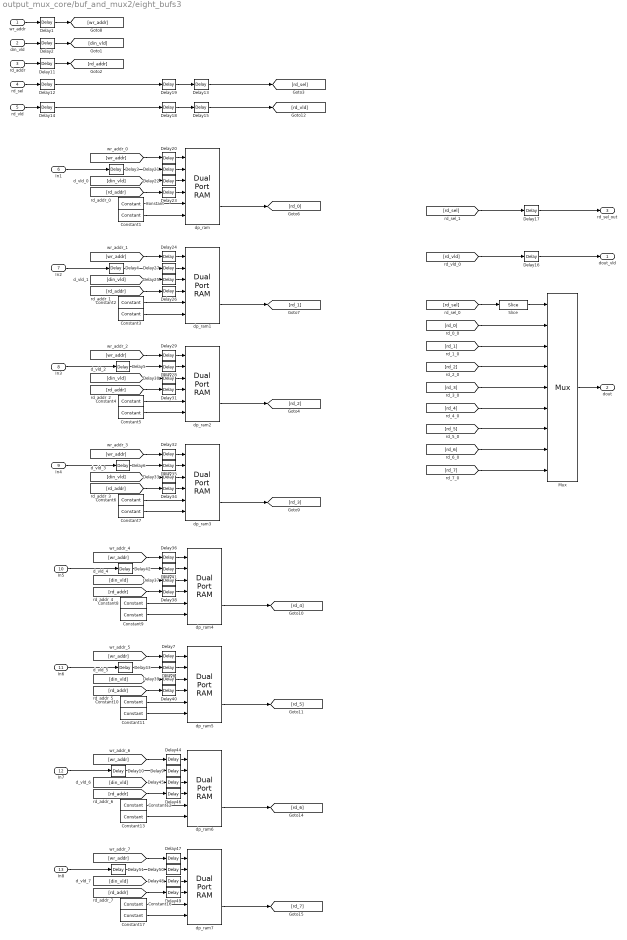
== system output_mux_core/buf_and_mux2/eight_bufs3 ==
  wr_addr : Inport
  din_vld : Inport  Port=2
  rd_addr : Inport  Port=3
  rd_sel : Inport  Port=4
  rd_vld : Inport  Port=5
  In1 : Inport  Port=6
  In2 : Inport  Port=7
  In3 : Inport  Port=8
  In4 : Inport  Port=9
  In5 : Inport  Port=10
  In6 : Inport  Port=11
  In7 : Inport  Port=12
  In8 : Inport  Port=13
  Constant{,2,4,6,8,10,12,16} (8 alike) : xbsIndex_r4/Constant  const=0  gui_display_data_type=Fixed-point  arith_type=Unsigned  n_bits=64  bin_pt=0  preci_type=Single  exp_width=8  frac_width=24  explicit_period=on  period=1  equ=P=C  opselect=C  inp2=PCIN>>17  opr=+  inp1=P  carry=CIN  dbl_ovrd=off  block_type=constant
  Constant{1,3,5,7,9,11,13,17} (8 alike) : xbsIndex_r4/Constant  const=0  gui_display_data_type=Boolean  arith_type=Boolean  n_bits=64  bin_pt=0  preci_type=Single  exp_width=8  frac_width=24  explicit_period=on  period=1  equ=P=C  opselect=C  inp2=PCIN>>17  opr=+  inp1=P  carry=CIN  dbl_ovrd=off  block_type=constant
  Delay{1..2,7,11..12,14,20,22..26,29..34,36..40,44..49} (29 alike) : xbsIndex_r4/Delay  rst=off  infoeditControl=Selection of Reset will increase slice count due to use of real FFs and instead of SRLs  en=off  latency=1  dbl_ovrd=off  reg_retiming=off  block_type=delay
  Delay{3..6,8..10,18..19,21,27..28,35,41..43,50..51} (18 alike) : xbsIndex_r4/Delay  rst=off  infoeditControl=Selection of Reset will increase slice count due to use of real FFs and instead of SRLs  en=off  latency=1  dbl_ovrd=off  reg_retiming=on  block_type=delay
  Delay13 : xbsIndex_r4/Delay  rst=off  infoeditControl=Selection of Reset will increase slice count due to use of real FFs and instead of SRLs  en=off  latency=3  dbl_ovrd=off  reg_retiming=on  block_type=delay
  Delay15 : xbsIndex_r4/Delay  rst=off  infoeditControl=Selection of Reset will increase slice count due to use of real FFs and instead of SRLs  en=off  latency=3  dbl_ovrd=off  reg_retiming=on  block_type=delay
  Delay16 : xbsIndex_r4/Delay  rst=off  infoeditControl=Selection of Reset will increase slice count due to use of real FFs and instead of SRLs  en=off  latency=2  dbl_ovrd=off  reg_retiming=off  block_type=delay
  Delay17 : xbsIndex_r4/Delay  rst=off  infoeditControl=Selection of Reset will increase slice count due to use of real FFs and instead of SRLs  en=off  latency=2  dbl_ovrd=off  reg_retiming=off  block_type=delay
  Mux : xbsIndex_r4/Mux  inputs=8  en=off  latency=2  precision=Full  arith_type=Unsigned  n_bits=16  bin_pt=14  quantization=Truncate  overflow=Wrap  dbl_ovrd=off  block_type=mux
  Slice : xbsIndex_r4/Slice  nbits=3  boolean_output=off  mode=Lower Bit Location + Width  bit1=0  base1=MSB of Input  bit0=0  base0=LSB of Input  dbl_ovrd=off  block_type=slice
  dp_ram{,1..7} (8 alike) : xbsIndex_r4/Dual Port RAM  depth=2^bram_depth  initVector=sin(pi*(0:15)/16)  distributed_mem=Block RAM  init_a=0  init_b=0  rst_a=off  rst_b=off  en_a=off  en_b=off  latency=3  write_mode_A=Read After Write  write_mode_B=Read After Write  dbl_ovrd=off  optimize=Speed  block_type=dpram
  dout_vld : Outport
  dout : Outport  Port=2
  rd_sel_out : Outport  Port=3
  wires:
  Delay50/1 -> dp_ram7/2
  Delay9/1 -> dp_ram6/2
  Delay49/1 -> dp_ram7/4
  Delay48/1 -> dp_ram7/3
  Delay47/1 -> dp_ram7/1
  Delay46/1 -> dp_ram6/4
  Delay45/1 -> dp_ram6/3
  Delay44/1 -> dp_ram6/1
  Delay8/1 -> dp_ram5/2
  Delay41/1 -> dp_ram4/2
  Delay40/1 -> dp_ram5/4
  Delay39/1 -> dp_ram5/3
  Delay7/1 -> dp_ram5/1
  Delay38/1 -> dp_ram4/4
  Delay37/1 -> dp_ram4/3
  Delay36/1 -> dp_ram4/1
  Delay35/1 -> dp_ram3/2
  Delay6/1 -> Delay35/1
  Delay34/1 -> dp_ram3/4
  Delay33/1 -> dp_ram3/3
  Delay32/1 -> dp_ram3/1
  Delay31/1 -> dp_ram2/4
  Delay30/1 -> dp_ram2/3
  Delay29/1 -> dp_ram2/1
  Delay28/1 -> dp_ram2/2
  Delay27/1 -> dp_ram1/2
  Delay26/1 -> dp_ram1/4
  Delay25/1 -> dp_ram1/3
  Delay24/1 -> dp_ram1/1
  Delay23/1 -> dp_ram/4
  Delay22/1 -> dp_ram/3
  Delay21/1 -> dp_ram/2
  Delay20/1 -> dp_ram/1
  Delay19/1 -> Delay13/1
  Delay18/1 -> Delay15/1
  Delay3/1 -> Delay21/1
  [rd_addr] -> Delay23/1
  [din_vld] -> Delay45/1
  [din_vld] -> Delay25/1
  Constant3/1 -> dp_ram1/6
  Constant2/1 -> dp_ram1/5
  In2/1 -> Delay4/1
  [rd_addr] -> Delay26/1
  [wr_addr] -> Delay24/1
  [wr_addr] -> Delay20/1
  [wr_addr] -> Delay32/1
  In5/1 -> Delay42/1
  [rd_addr] -> Delay49/1
  Constant5/1 -> dp_ram2/6
  Constant/1 -> dp_ram/5
  In7/1 -> Delay10/1
  [wr_addr] -> Delay29/1
  [wr_addr] -> Delay36/1
  In8/1 -> Delay51/1
  In3/1 -> Delay5/1
  Constant9/1 -> dp_ram4/6
  Constant6/1 -> dp_ram3/5
  In6/1 -> Delay43/1
  Constant16/1 -> dp_ram7/5
  [wr_addr] -> Delay47/1
  Delay5/1 -> Delay28/1
  [rd_addr] -> Delay31/1
  Delay10/1 -> Delay9/1
  [rd_addr] -> Delay34/1
  In1/1 -> Delay3/1
  [rd_addr] -> Delay40/1
  [din_vld] -> Delay37/1
  [din_vld] -> Delay48/1
  Delay43/1 -> Delay8/1
  [din_vld] -> Delay30/1
  Constant8/1 -> dp_ram4/5
  Constant12/1 -> dp_ram6/5
  Constant4/1 -> dp_ram2/5
  [rd_addr] -> Delay38/1
  Constant10/1 -> dp_ram5/5
  [din_vld] -> Delay33/1
  Delay42/1 -> Delay41/1
  Constant13/1 -> dp_ram6/6
  Constant11/1 -> dp_ram5/6
  In4/1 -> Delay6/1
  Constant7/1 -> dp_ram3/6
  [rd_addr] -> Delay46/1
  Delay51/1 -> Delay50/1
  Delay4/1 -> Delay27/1
  [din_vld] -> Delay39/1
  [din_vld] -> Delay22/1
  [wr_addr] -> Delay7/1
  Constant17/1 -> dp_ram7/6
  [wr_addr] -> Delay44/1
  Constant1/1 -> dp_ram/6
  wr_addr/1 -> Delay1/1
  Delay1/1 -> [wr_addr]
  din_vld/1 -> Delay2/1
  Delay2/1 -> [din_vld]
  rd_addr/1 -> Delay11/1
  Delay11/1 -> [rd_addr]
  rd_sel/1 -> Delay12/1
  Delay12/1 -> Delay19/1
  Delay13/1 -> [rd_sel]
  dp_ram/2 -> [rd_0]
  dp_ram1/2 -> [rd_1]
  dp_ram2/2 -> [rd_2]
  dp_ram3/2 -> [rd_3]
  dp_ram4/2 -> [rd_4]
  dp_ram5/2 -> [rd_5]
  dp_ram6/2 -> [rd_6]
  dp_ram7/2 -> [rd_7]
  [rd_3] -> Mux/5
  [rd_6] -> Mux/8
  [rd_7] -> Mux/9
  [rd_sel] -> Slice/1
  [rd_4] -> Mux/6
  [rd_5] -> Mux/7
  [rd_0] -> Mux/2
  [rd_2] -> Mux/4
  [rd_1] -> Mux/3
  Mux/1 -> dout/1
  rd_vld/1 -> Delay14/1
  Delay15/1 -> [rd_vld]
  Delay14/1 -> Delay18/1
  [rd_vld] -> Delay16/1
  Delay16/1 -> dout_vld/1
  [rd_sel] -> Delay17/1
  Delay17/1 -> rd_sel_out/1
  Slice/1 -> Mux/1
